simulink model "datacapture_model"  (R2017b)
settings: Solver=VariableStepAuto  StartTime=0.0  StopTime=inf  RelTol=1e-3
libraries: hdlverifier_fpga_reader x1
settings Model: Creator=Faseeh  LastModifiedBy=Faseeh

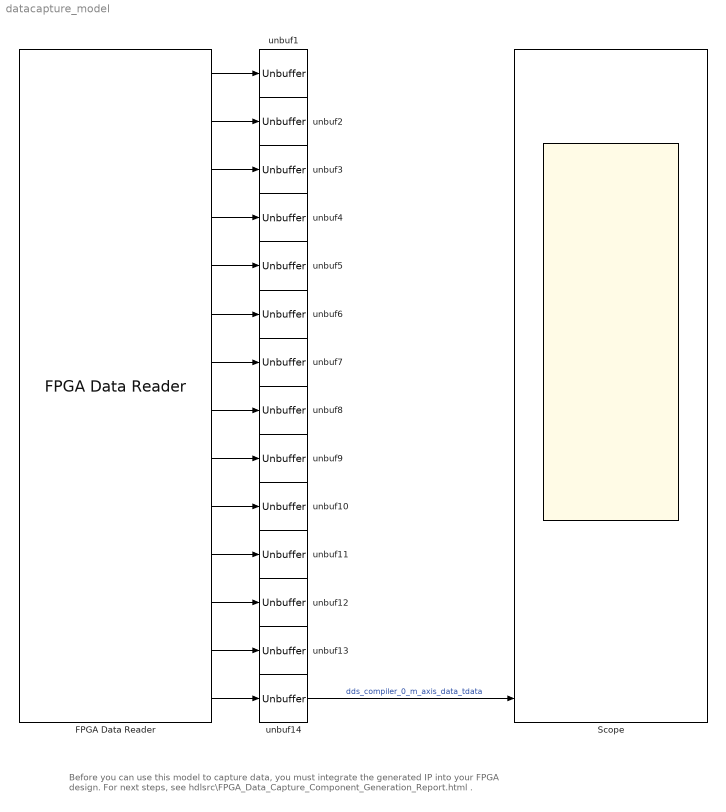
== system datacapture_model ==
  note: Before you can use this model to capture data, you must integrate the generated IP into your FPGA design.
      | For next steps, see hdlsrc\FPGA_Data_Capture_Component_Generation_Report.html .
  FPGA Data Reader : hdlverifier_fpga_reader/FPGA Data Reader  SampleTime=2048  FPGAVendor=Xilinx  SamplesPerFrame=2048  TriggerPosition=0  TimeOut=10  TriggerConditionStr="[false,\"0\",false,\"Low\",false,\"Low\",false,\"Low\",false,\"Low\",false,\"Low\",false,\"Low\",false,\"Low\",false,\"Low\",false,\"0\",false,\"0\",false,\"Low\",false,\"Low\",false,\"0\",\"and\"]"  DataTypeStr="[\"uint16\",\"boolean\",\"boolean\",\"boolean\",\"boolean\",\"boolean\",\"boolean\",\"boolean\",\"boolean\",\"uint16\",\"uint16\",\"boolean\",\"boolean\",\"uint8\"]"  BitWidth="[16   1   1   1   1   1   1   1   1  16  16   1   1   8]"  SignalNames={'m_axis_data_tdata','xfft_0_s_axis_config_tready','xfft_0_s_axis_data_tready','xfft_0_event_data_out_channel_halt','xfft_0_event_data_in_channel_halt','xfft_0_event_status_channel_halt','xfft_0_event_tlast_missing','xfft_0_event_tlast_unexpected','xfft_0_event_frame_started','xfft_0_m_axis_data_tdata','xfft_0_m_axis_data_tuser','xfft_0_m_axis_data_tvalid','xfft_0_m_axis_data_tlast','dds_compiler_0_m_axis_data_tdata'}  IsSignalTrigger="[1  1  1  1  1  1  1  1  1  1  1  1  1  1]"  IsSignalData="[1  1  1  1  1  1  1  1  1  1  1  1  1  1]"  JTAGCableName=auto  JTAGChainPosition=0  IRLengthBefore=0  IRLengthAfter=0  TckFrequency=15
  Scope : Scope  NumInputPorts=14
  unbuf{1..14} (14 alike) : Unbuffer
  wires:
  FPGA Data Reader/1 -> unbuf1/1
  FPGA Data Reader/2 -> unbuf2/1
  FPGA Data Reader/3 -> unbuf3/1
  FPGA Data Reader/4 -> unbuf4/1
  FPGA Data Reader/5 -> unbuf5/1
  FPGA Data Reader/6 -> unbuf6/1
  FPGA Data Reader/7 -> unbuf7/1
  FPGA Data Reader/8 -> unbuf8/1
  FPGA Data Reader/9 -> unbuf9/1
  FPGA Data Reader/10 -> unbuf10/1
  FPGA Data Reader/11 -> unbuf11/1
  FPGA Data Reader/12 -> unbuf12/1
  FPGA Data Reader/13 -> unbuf13/1
  FPGA Data Reader/14 -> unbuf14/1
  unbuf14/1 -> Scope/14  "dds_compiler_0_m_axis_data_tdata"
